simulink model "ControlWillyBCangulo"  (R2021b)
settings: Solver=FixedStepAuto  StartTime=0.0  StopTime=10.0  RelTol=1e-3  EnableMultiTasking=on
StartFcn:
  | dg = 0.2
model workspace (MAT data in the model file):
  dg = 0.2
settings Model: ExtModeTrigDuration=2  Creator=ferna  LastModifiedBy=ferna
settings OptimizationCC: EnhancedBackFolding=on  PassReuseOutputArgsAs=Individual arguments  ZeroExternalMemoryAtStartup=off  ZeroInternalMemoryAtStartup=off  MaxStackSize=64  OptimizeBlockOrder=speed  DifferentSizesBufferReuse=on  EfficientTunableParamExpr=on
settings DebuggingCC: ParameterTunabilityLossMsg=error
settings HardwareCC: ProdBitPerInt=16  ProdBitPerPointer=16  ProdBitPerSizeT=16  ProdBitPerPtrDiffT=16  ProdLargestAtomicFloat=None  ProdWordSize=8  ProdHWDeviceType=Atmel->AVR
settings SFSimCC: MATLABDynamicMemAlloc=off
settings RTWCC: Description=Embedded Coder  SystemTargetFile=ert.tlc  HardwareBoard=Arduino Mega 2560  TemplateMakefile=ert_default_tmf  Toolchain=Arduino AVR  BuildConfiguration=Faster Runs
settings CodeAppCC: ForceParamTrailComments=on  IgnoreCustomStorageClasses=off  OperatorAnnotations=on  SimulinkDataObjDesc=on  SFDataObjDesc=on  InsertBlockDesc=on
settings ERTTargetCC: SupportContinuousTime=on  SupportVariableSizeSignals=on  ExtModeTransport=3  ExtModeStaticAlloc=on  ExtModeStaticAllocSize=2048  ExtModeMexFile=ext_xcp  ExtModeIntrfLevel=Level2 - Open

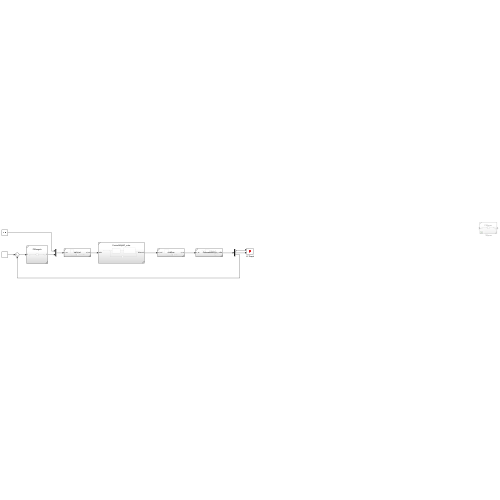
[thumbnail: Simulink's stored preview of the top-level diagram]
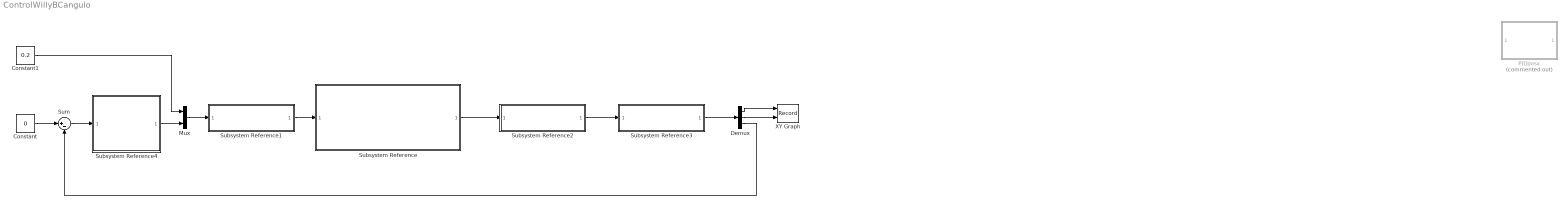
== system ControlWillyBCangulo ==
  Constant : Constant  Value=0  SampleTime=0.01
  Constant1 : Constant  Value=0.2
  Demux : Demux  Outputs=3
  Mux : Mux  Inputs=2
  PIDposx : Subsystem  Commented=on  ReferencedSubsystem=PIDposx
  Subsystem Reference : Subsystem  ReferencedSubsystem=ControlWillyBC_subs
  Subsystem Reference1 : Subsystem  ReferencedSubsystem=vw2vivd
  Subsystem Reference2 : Subsystem  ReferencedSubsystem=vivd2vw
  Subsystem Reference3 : Subsystem  ReferencedSubsystem=OdometriaWilly
  Subsystem Reference4 : Subsystem  ReferencedSubsystem=PIDangulo
  Sum : Sum  Inputs=|+-
  XY Graph : Record  FileSettingsInternal="{\"entries\":[{\"content\":{\"excelSettings\":{\"content\":{},\"type\":\"Streamout.ExcelSettings\"}},\"type\":\"Streamout.FileSettingStorage\",\"uuid\":\"8aa3d5bb-48ff-4e2f-b3f8-bbff7ebf77b2\"}],\"packageUris\":[\"http://schema.mathworks.com/mf0/streamout_blocks/R2020a\"],\"version\":\"1.0\"}"  Layout=[1 1]  SignalsInternal="{\"entries\":[{\"content\":{\"signals\":[{\"content\":{\"blockPath\":[\"ControlWillyBCangulo/XY Graph\"],\"channel\":[],\"dimensions\":[1],\"domain\":\"ControlWillyBCangulo/XY Graph\",\"lineColor\":\"#a2142f\",\"plots\":[],\"port\":1,\"sid\":[\"\"],\"signalID\":58,\"signalName\":\"Demux:1\"},\"type\":\"RecordBlkView.Signal\",\"uuid\":\"bb90c503-28a0-4acb-8ceb-3579370addd3\"},{\"content\":{\"blockPath\":[\"ControlWillyBCangulo/XY Graph\"],\"channel\":[],\"dimensions\":[1],\"domain\":\"ControlWillyBCangulo/XY Graph\",\"lineColor\":\"#139fff\",\"plots\":[],\"port\":2,\"sid\":[\"\"],\"signalID\":62,\"signalName\":\"Demux:2\"},\"type\":\"RecordBlkView.Signal\",\"uuid\":\"cc9aa5d6-0433-4af7-b739-c68da0e3ce7c\"}]},\"type\":\"RecordBlkView.InputSignals\",\"uuid\":\"d095def6-9339-4d58-9688-10e11b1f8184\"}],\"packageUris\":[\"http://schema.mathworks.com/mf0/streamout_blocks/R2020a\"],\"version\":\"1.0\"}"  VisualizationBindings="{\"xyplotplugin\":{\"info\":[{\"series\":[],\"subplotID\":1}]}}"  CompatibilityTag=XY
  wires:
  Subsystem Reference1/1 -> Subsystem Reference/1
  Subsystem Reference2/1 -> Subsystem Reference3/1
  Subsystem Reference3/1 -> Demux/1
  Subsystem Reference/1 -> Subsystem Reference2/1
  Demux/2 -> XY Graph/2
  Demux/1 -> XY Graph/1
  Mux/1 -> Subsystem Reference1/1
  Subsystem Reference4/1 -> Mux/2
  Sum/1 -> Subsystem Reference4/1
  Constant/1 -> Sum/1
  Demux/3 -> Sum/2
  Constant1/1 -> Mux/1
